simulink model "SolarWithBoost"  (R2021a)
settings: Solver=VariableStepAuto  StartTime=0.0  StopTime=1  FixedStep=0.1  RelTol=1e-3
libraries: spsSeriesRLCBranchLib x4, spsVoltageMeasurementLib x2, spsDiodeLib x1, spsMosfetLib x1, spsCurrentMeasurementLib x1, spsPVArrayLib x1, spspowerguiLib x1
settings Model: Creator=Б.Шинэхүү  LastModifiedBy=Б.Шинэхүү

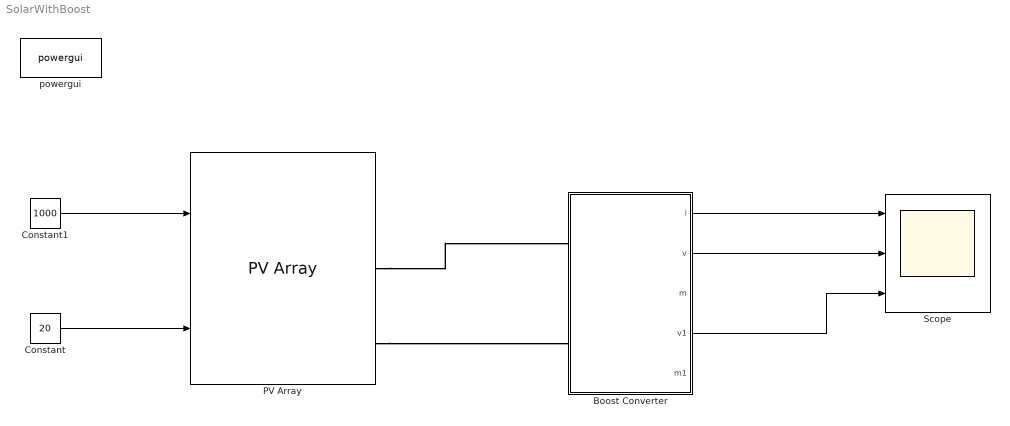
== system SolarWithBoost ==
  Boost Converter : Subsystem
  Constant : Constant  Value=20
  Constant1 : Constant  Value=1000
  PV Array : spsPVArrayLib/PV Array  Npar=2  Nser=1  PlotType=array @ 1000 W/m2 & specified temperatures  S_vec="[ 1000  500  100 ]"  Temp_C_vec="[ 45 20  ]"  ModuleName=User-defined  PlotWhenSelected=off  Pm=240.5352  Ncell=64  Voc=21.9  Isc=14.1  Vm=18.3  Im=13.144  beta_Voc_pc=-0.36099  alpha_Isc_pc=0.102  beta_Voc=-0.079057  alpha_Isc=0.014382  IL=14.1141  I0=5.1873e-10  nI=0.55489  Rsh=64.4292  Rs=0.064327  RobustModel=off  RobustCellTemperature=313.3991  BAL=on  Tc=1e-6  Tfilter=5e-5
  Scope : Scope  NumInputPorts=3
  powergui : spspowerguiLib/powergui  Priority=1  SimulationMode=Continuous  SampleTime=1e-6  frequency=60  Iterations=50  frequencyindice=0  Pbase=100e6  ErrMax=1e-4  UnitsV=kV  UnitsW=MW  buscounter=0  FunctionMessages=off  echomessages=off  EnableUseOfTLC=off  CurrentSourceSwitches=off  DisableSnubberDevices=off  DisableRonSwitches=off  DisableVfSwitches=off  DisplayEquations=off  AutomaticDiscreteSolvers=off  SolverType=Tustin/Backward Euler (TBE)  Interpol=off  ExternalGateDelay=off  methode=off  Ts=100  x0status=blocks  SPID=on  SwTol=0  HookPort=off  NonlinearTolerance=1e-4  nMaxIteration=100  ContinueOnMaxIteration=off  RestoreLinks=warning  ResistiveCurrentMeasurement=off  Frange=[0:2:500]  Ylog=off  Xlog=on  ShowGrid=off  save=off  variable=ZData  structure=0  ZoomFFT=off  StartTime=0.0  cycles=1  DisplayStyle=1  fundamental=60  FreqAxis=off  MaxFrequency=1000  frequencyindicesteady=1  RmsSteady=1  display=off
  wires:
  Constant1/1 -> PV Array/1
  Constant/1 -> PV Array/2
  Boost Converter/1(i) -> Scope/1
  Boost Converter/2(v) -> Scope/2
  Boost Converter/4(v1) -> Scope/3
  connections:
  PV Array/RConn1 -- Boost Converter/LConn1
  PV Array/RConn2 -- Boost Converter/LConn2

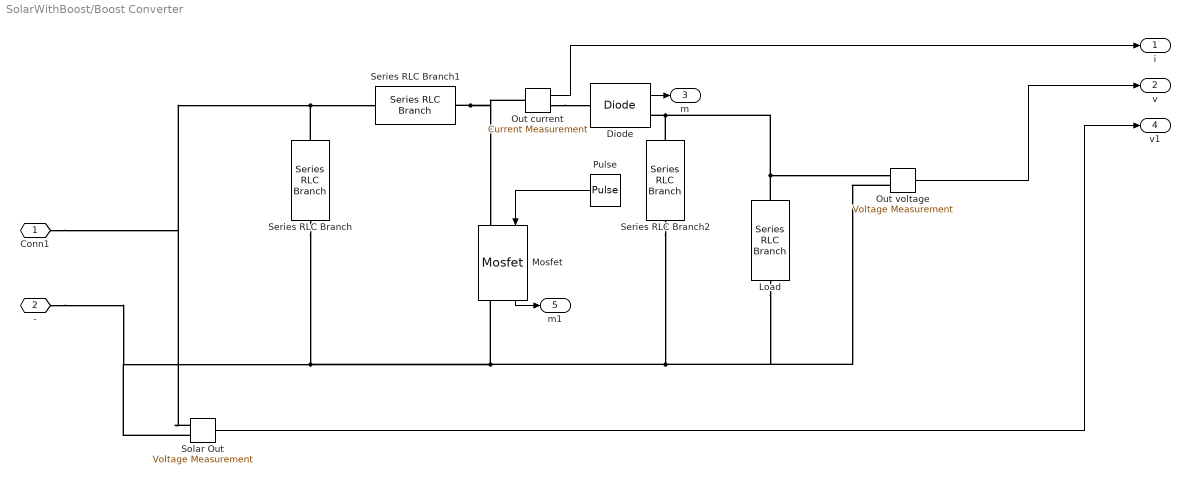
== system SolarWithBoost/Boost Converter ==
  Diode : spsDiodeLib/Diode  Ron=0.001  Lon=0  Vf=0.8  IC=0  UseSnubber=0  Rs=500  Cs=250e-9  Measurements=on
  Load : spsSeriesRLCBranchLib/Series RLC Branch  LConnTagsString=__new0  RConnTagsString=__new0  BranchType=R  Resistance=10  Inductance=5e-3  SetiL0=off  InitialCurrent=0  Capacitance=100e-3  Setx0=off  InitialVoltage=0  Measurements=None
  Mosfet : spsMosfetLib/Mosfet  Ron=0.1  Lon=0  Rd=0.01  Vfd=0  IC=0  Rs=1e5  Cs=inf  Measurements=on
  Out current : spsCurrentMeasurementLib/Current Measurement  PhasorSimulation=off  OutputType=Complex  PSBequivalent=0
  Out voltage : spsVoltageMeasurementLib/Voltage Measurement  PhasorSimulation=off  OutputType=Complex  PSBequivalent=0
  Pulse : DiscretePulseGenerator  PulseType=Time based  Period=1/25000  PulseWidth=8.7
  Series RLC Branch : spsSeriesRLCBranchLib/Series RLC Branch  LConnTagsString=__new0  RConnTagsString=__new0  BranchType=C  Resistance=1  Inductance=1e-3  SetiL0=off  InitialCurrent=0  Capacitance=10e-6  Setx0=off  InitialVoltage=0  Measurements=None
  Series RLC Branch1 : spsSeriesRLCBranchLib/Series RLC Branch  LConnTagsString=__new0  RConnTagsString=__new0  BranchType=L  Resistance=0.000001  Inductance=0.000013  SetiL0=off  InitialCurrent=0  Capacitance=100e-6  Setx0=off  InitialVoltage=0  Measurements=None
  Series RLC Branch2 : spsSeriesRLCBranchLib/Series RLC Branch  LConnTagsString=__new0  RConnTagsString=__new0  BranchType=C  Resistance=0.000001  Inductance=5e-3  SetiL0=off  InitialCurrent=0  Capacitance=0.00006  Setx0=off  InitialVoltage=0  Measurements=None
  Solar Out : spsVoltageMeasurementLib/Voltage Measurement  PhasorSimulation=off  OutputType=Complex  PSBequivalent=0
  Conn1 : PMIOPort  Side=Left
  - : PMIOPort  Port=2  Side=Left
  i : Outport
  v : Outport  Port=2
  m : Outport  Port=3
  v1 : Outport  Port=4
  m1 : Outport  Port=5
  wires:
  Out voltage/1 -> v/1
  Pulse/1 -> Mosfet/1
  Solar Out/1 -> v1/1
  Out current/1 -> i/1
  Diode/1 -> m/1
  Mosfet/1 -> m1/1
  connections:
  Series RLC Branch1/LConn1 -- Mosfet/LConn1 -- Out current/LConn1
  Series RLC Branch/LConn1 -- Conn1/RConn1 -- Solar Out/LConn1 -- Series RLC Branch1/RConn1
  Series RLC Branch/RConn1 -- -/RConn1 -- Solar Out/LConn2 -- Mosfet/RConn1 -- Series RLC Branch2/LConn1 -- Out voltage/LConn2 -- Load/LConn1
  Out current/RConn1 -- Diode/LConn1
  Load/RConn1 -- Series RLC Branch2/RConn1 -- Diode/RConn1 -- Out voltage/LConn1
